simulink subsystem "segment_24S2P"  (R2019b)
settings: Solver=VariableStepAuto  StartTime=0.0  StopTime=10.0  RelTol=1e-3
values from neighbouring files (symbols this model uses):
  cell_prop = struct    [data_load.m]    (also in extend_model_ini.m = data_load('Cell_data.xlsx'))
libraries: fl_lib x44
settings Model: Creator=ZHOU Jinhan  LastModifiedBy=ZHOU Jinhan

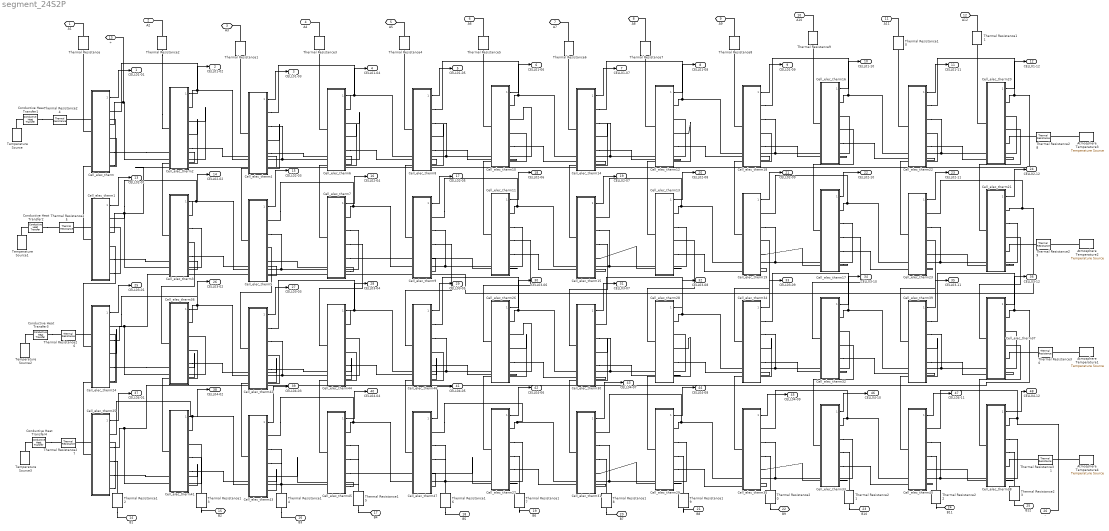
== system segment_24S2P ==
  Atmosphere Temperature{1..4} (4 alike) : fl_lib/Thermal/Thermal Sources/Temperature Source  temperature=cell_prop.T_ext K
      settings: SourceProductName=Simscape
  Cell_elec_therm{,1..47} (48 alike) : Subsystem  ReferencedSubsystem=Cell_elec_therm
  Conductive Heat Transfer{1..4} (4 alike) : fl_lib/Thermal/Thermal Elements/Conductive Heat Transfer  area=0.1 m^2  thickness=0.1 m  th_cond=cell_prop.CFM*0.56657223796 W/(m*K)  T_specify=off  T_priority=None  T=0 K  T_nominal_specify=off  T_nominal_unit=K  T_nominal_value=1  Q_specify=off  Q_priority=None  Q=0 W  Q_nominal_specify=off  Q_nominal_unit=W  Q_nominal_value=1
      settings: SourceProductName=Simscape
  Temperature Source{,1..3} (4 alike) : fl_lib/Thermal/Thermal Sources/Temperature Source  temperature=cell_prop.T_ext K
      settings: SourceProductName=Simscape
  Thermal Resistance{,1..23} (24 alike) : fl_lib/Thermal/Thermal Elements/Thermal Resistance  resistance=1/cell_prop.cell_height*cell_prop.cell_width*cell_prop.wall*0.007874*0.4773 K/W  T_specify=off  T_priority=None  T=0 K  T_nominal_specify=off  T_nominal_unit=K  T_nominal_value=1  Q_specify=off  Q_priority=None  Q=0 W  Q_nominal_specify=off  Q_nominal_unit=W  Q_nominal_value=1
      settings: SourceProductName=Simscape  SourceProductBaseCode=SS
  Thermal Resistance{24..31} (8 alike) : fl_lib/Thermal/Thermal Elements/Thermal Resistance  resistance=1/cell_prop.cell_height*cell_prop.cell_length*cell_prop.wall*0.007874*0.4773 K/W  T_specify=off  T_priority=None  T=0 K  T_nominal_specify=off  T_nominal_unit=K  T_nominal_value=1  Q_specify=off  Q_priority=None  Q=0 W  Q_nominal_specify=off  Q_nominal_unit=W  Q_nominal_value=1
      settings: SourceProductName=Simscape  SourceProductBaseCode=SS
  A1 : PMIOPort  Side=Left
  A2 : PMIOPort  Port=2  Side=Left
  A3 : PMIOPort  Port=3  Side=Left
  A4 : PMIOPort  Port=4  Side=Left
  A5 : PMIOPort  Port=5  Side=Left
  A6 : PMIOPort  Port=6  Side=Left
  A7 : PMIOPort  Port=7  Side=Left
  A8 : PMIOPort  Port=8  Side=Left
  A9 : PMIOPort  Port=9  Side=Left
  A10 : PMIOPort  Port=10  Side=Left
  A11 : PMIOPort  Port=11  Side=Left
  A12 : PMIOPort  Port=12  Side=Left
  + : PMIOPort  Port=13  Side=Left
  B1 : PMIOPort  Port=14  Side=Left
  B2 : PMIOPort  Port=15  Side=Left
  B3 : PMIOPort  Port=16  Side=Left
  B4 : PMIOPort  Port=17  Side=Left
  B5 : PMIOPort  Port=18  Side=Left
  B6 : PMIOPort  Port=19  Side=Left
  B7 : PMIOPort  Port=20  Side=Left
  B8 : PMIOPort  Port=21  Side=Left
  B9 : PMIOPort  Port=22  Side=Left
  B10 : PMIOPort  Port=23  Side=Left
  B11 : PMIOPort  Port=24  Side=Left
  B12 : PMIOPort  Port=25  Side=Left
  - : PMIOPort  Port=26  Side=Left
  CELL01-01 : Outport
  CELL01-02 : Outport  Port=2
  CELL01-03 : Outport  Port=3
  CELL01-04 : Outport  Port=4
  CELL01-05 : Outport  Port=5
  CELL01-06 : Outport  Port=6
  CELL01-07 : Outport  Port=7
  CELL01-08 : Outport  Port=8
  CELL01-09 : Outport  Port=9
  CELL01-10 : Outport  Port=10
  CELL01-11 : Outport  Port=11
  CELL01-12 : Outport  Port=12
  CELL02-01 : Outport  Port=13
  CELL02-02 : Outport  Port=14
  CELL02-03 : Outport  Port=15
  CELL02-04 : Outport  Port=16
  CELL02-05 : Outport  Port=17
  CELL02-06 : Outport  Port=18
  CELL02-07 : Outport  Port=19
  CELL02-08 : Outport  Port=20
  CELL02-09 : Outport  Port=21
  CELL02-10 : Outport  Port=22
  CELL02-11 : Outport  Port=23
  CELL02-12 : Outport  Port=24
  CELL03-01 : Outport  Port=25
  CELL03-02 : Outport  Port=26
  CELL03-03 : Outport  Port=27
  CELL03-04 : Outport  Port=28
  CELL03-05 : Outport  Port=29
  CELL03-06 : Outport  Port=30
  CELL03-07 : Outport  Port=31
  CELL03-08 : Outport  Port=32
  CELL03-09 : Outport  Port=33
  CELL03-10 : Outport  Port=34
  CELL03-11 : Outport  Port=35
  CELL03-12 : Outport  Port=36
  CELL04-01 : Outport  Port=37
  CELL04-02 : Outport  Port=38
  CELL04-03 : Outport  Port=39
  CELL04-04 : Outport  Port=40
  CELL04-05 : Outport  Port=41
  CELL04-06 : Outport  Port=42
  CELL04-07 : Outport  Port=43
  CELL04-08 : Outport  Port=44
  CELL04-09 : Outport  Port=45
  CELL04-10 : Outport  Port=46
  CELL04-11 : Outport  Port=47
  CELL04-12 : Outport  Port=48
  wires:
  Cell_elec_therm3/1 -> CELL02-02/1
  Cell_elec_therm26/1 -> CELL03-06/1
  Cell_elec_therm7/1 -> CELL02-04/1
  Cell_elec_therm28/1 -> CELL03-08/1
  Cell_elec_therm10/1 -> CELL01-06/1
  Cell_elec_therm17/1 -> CELL02-10/1
  Cell_elec_therm32/1 -> CELL03-10/1
  Cell_elec_therm45/1 -> CELL04-04/1
  Cell_elec_therm1/1 -> CELL02-01/1
  Cell_elec_therm9/1 -> CELL02-05/1
  Cell_elec_therm22/1 -> CELL01-11/1
  Cell_elec_therm21/1 -> CELL02-12/1
  Cell_elec_therm15/1 -> CELL02-07/1
  Cell_elec_therm23/1 -> CELL02-11/1
  Cell_elec_therm/1 -> CELL01-01/1
  Cell_elec_therm13/1 -> CELL02-08/1
  Cell_elec_therm20/1 -> CELL01-12/1
  Cell_elec_therm12/1 -> CELL01-08/1
  Cell_elec_therm14/1 -> CELL01-07/1
  Cell_elec_therm18/1 -> CELL01-09/1
  Cell_elec_therm31/1 -> CELL04-07/1
  Cell_elec_therm16/1 -> CELL01-10/1
  Cell_elec_therm19/1 -> CELL02-09/1
  Cell_elec_therm42/1 -> CELL03-03/1
  Cell_elec_therm2/1 -> CELL01-02/1
  Cell_elec_therm25/1 -> CELL04-01/1
  Cell_elec_therm40/1 -> CELL04-11/1
  Cell_elec_therm24/1 -> CELL03-01/1
  Cell_elec_therm27/1 -> CELL04-06/1
  Cell_elec_therm47/1 -> CELL04-05/1
  Cell_elec_therm41/1 -> CELL04-02/1
  Cell_elec_therm46/1 -> CELL03-05/1
  Cell_elec_therm30/1 -> CELL03-07/1
  Cell_elec_therm43/1 -> CELL04-03/1
  Cell_elec_therm33/1 -> CELL04-10/1
  Cell_elec_therm29/1 -> CELL04-08/1
  Cell_elec_therm44/1 -> CELL03-04/1
  Cell_elec_therm37/1 -> CELL03-12/1
  Cell_elec_therm35/1 -> CELL04-09/1
  Cell_elec_therm38/1 -> CELL04-12/1
  Cell_elec_therm34/1 -> CELL03-09/1
  Cell_elec_therm39/1 -> CELL03-11/1
  Cell_elec_therm36/1 -> CELL03-02/1
  Cell_elec_therm6/1 -> CELL01-04/1
  Cell_elec_therm5/1 -> CELL02-03/1
  Cell_elec_therm8/1 -> CELL01-05/1
  Cell_elec_therm11/1 -> CELL02-06/1
  Cell_elec_therm4/1 -> CELL01-03/1
  connections:
  Cell_elec_therm37/RConn1 -- Cell_elec_therm25/RConn2 -- Cell_elec_therm41/RConn2 -- Cell_elec_therm39/RConn1
  Cell_elec_therm12/RConn1 -- Cell_elec_therm16/RConn2 -- Cell_elec_therm18/RConn2 -- Cell_elec_therm14/RConn1
  Cell_elec_therm13/RConn1 -- Cell_elec_therm15/RConn1 -- Cell_elec_therm17/RConn2 -- Cell_elec_therm19/RConn2
  Cell_elec_therm41/RConn1 -- Cell_elec_therm25/RConn1 -- Cell_elec_therm45/RConn2 -- Cell_elec_therm43/RConn2
  Cell_elec_therm28/RConn1 -- Cell_elec_therm34/RConn2 -- Cell_elec_therm32/RConn2 -- Cell_elec_therm30/RConn1
  Cell_elec_therm/RConn2 -- Cell_elec_therm2/RConn2 -- +/RConn1
  Cell_elec_therm5/RConn2 -- Cell_elec_therm3/RConn1 -- Cell_elec_therm1/RConn1 -- Cell_elec_therm7/RConn2
  Cell_elec_therm18/RConn1 -- Cell_elec_therm16/RConn1 -- Cell_elec_therm20/RConn2 -- Cell_elec_therm22/RConn2
  Cell_elec_therm37/RConn2 -- Cell_elec_therm32/RConn1 -- Cell_elec_therm34/RConn1 -- Cell_elec_therm39/RConn2
  Cell_elec_therm9/RConn2 -- Cell_elec_therm5/RConn1 -- Cell_elec_therm7/RConn1 -- Cell_elec_therm11/RConn2
  Cell_elec_therm17/RConn1 -- Cell_elec_therm19/RConn1 -- Cell_elec_therm21/RConn2 -- Cell_elec_therm23/RConn2
  Cell_elec_therm47/RConn2 -- Cell_elec_therm43/RConn1 -- Cell_elec_therm45/RConn1 -- Cell_elec_therm27/RConn2
  Cell_elec_therm1/RConn2 -- Cell_elec_therm20/RConn1 -- Cell_elec_therm22/RConn1 -- Cell_elec_therm3/RConn2
  Cell_elec_therm42/RConn2 -- Cell_elec_therm44/RConn2 -- Cell_elec_therm24/RConn1 -- Cell_elec_therm36/RConn1
  Cell_elec_therm27/RConn1 -- Cell_elec_therm29/RConn2 -- Cell_elec_therm31/RConn2 -- Cell_elec_therm47/RConn1
  Cell_elec_therm35/RConn2 -- Cell_elec_therm31/RConn1 -- Cell_elec_therm29/RConn1 -- Cell_elec_therm33/RConn2
  Cell_elec_therm2/RConn1 -- Cell_elec_therm6/RConn2 -- Cell_elec_therm4/RConn2 -- Cell_elec_therm/RConn1
  Cell_elec_therm6/RConn1 -- Cell_elec_therm10/RConn2 -- Cell_elec_therm8/RConn2 -- Cell_elec_therm4/RConn1
  Cell_elec_therm33/RConn1 -- Cell_elec_therm38/RConn2 -- Cell_elec_therm40/RConn2 -- Cell_elec_therm35/RConn1
  Cell_elec_therm21/RConn1 -- Cell_elec_therm36/RConn2 -- Cell_elec_therm24/RConn2 -- Cell_elec_therm23/RConn1
  Cell_elec_therm10/RConn1 -- Cell_elec_therm12/RConn2 -- Cell_elec_therm14/RConn2 -- Cell_elec_therm8/RConn1
  Cell_elec_therm11/RConn1 -- Cell_elec_therm9/RConn1 -- Cell_elec_therm13/RConn2 -- Cell_elec_therm15/RConn2
  Cell_elec_therm40/RConn1 -- Cell_elec_therm38/RConn1 -- -/RConn1
  Cell_elec_therm28/RConn2 -- Cell_elec_therm46/RConn1 -- Cell_elec_therm26/RConn1 -- Cell_elec_therm30/RConn2
  Cell_elec_therm46/RConn2 -- Cell_elec_therm42/RConn1 -- Cell_elec_therm44/RConn1 -- Cell_elec_therm26/RConn2
  Thermal Resistance3/RConn1 -- A4/RConn1
  Cell_elec_therm12/LConn1 -- Thermal Resistance7/LConn1
  Cell_elec_therm7/RConn4 -- Cell_elec_therm9/RConn5
  Cell_elec_therm3/RConn4 -- Cell_elec_therm5/RConn5
  Cell_elec_therm17/RConn5 -- Cell_elec_therm19/RConn4
  Cell_elec_therm7/RConn5 -- Cell_elec_therm5/RConn4
  Cell_elec_therm10/LConn1 -- Thermal Resistance5/LConn1
  Cell_elec_therm45/LConn1 -- Cell_elec_therm44/RConn3
  Cell_elec_therm15/RConn3 -- Cell_elec_therm30/LConn1
  Cell_elec_therm10/RConn4 -- Cell_elec_therm14/RConn5
  Cell_elec_therm21/RConn5 -- Cell_elec_therm23/RConn4
  Thermal Resistance23/LConn1 -- B12/RConn1
  Cell_elec_therm13/RConn5 -- Cell_elec_therm15/RConn4
  Cell_elec_therm46/RConn4 -- Cell_elec_therm26/RConn5
  Cell_elec_therm22/RConn4 -- Cell_elec_therm20/RConn5
  Cell_elec_therm6/RConn4 -- Cell_elec_therm8/RConn5
  Cell_elec_therm33/LConn1 -- Cell_elec_therm32/RConn3
  Cell_elec_therm21/LConn1 -- Cell_elec_therm20/RConn3
  Cell_elec_therm29/LConn1 -- Cell_elec_therm28/RConn3
  Cell_elec_therm16/RConn4 -- Cell_elec_therm22/RConn5
  Cell_elec_therm23/LConn1 -- Cell_elec_therm22/RConn3
  Thermal Resistance2/LConn1 -- Cell_elec_therm2/LConn1
  Cell_elec_therm17/RConn3 -- Cell_elec_therm32/LConn1
  Cell_elec_therm1/LConn1 -- Cell_elec_therm/RConn3
  Cell_elec_therm32/RConn4 -- Cell_elec_therm39/RConn5
  Cell_elec_therm39/RConn4 -- Cell_elec_therm37/RConn5
  Cell_elec_therm14/RConn4 -- Cell_elec_therm12/RConn5
  Atmosphere Temperature4/LConn1 -- Thermal Resistance31/LConn1
  Cell_elec_therm37/LConn1 -- Cell_elec_therm21/RConn3
  Cell_elec_therm44/RConn4 -- Cell_elec_therm46/RConn5
  Cell_elec_therm17/LConn1 -- Cell_elec_therm16/RConn3
  Cell_elec_therm13/LConn1 -- Cell_elec_therm12/RConn3
  Cell_elec_therm15/LConn1 -- Cell_elec_therm14/RConn3
  Thermal Resistance9/RConn1 -- A10/RConn1
  Cell_elec_therm9/RConn3 -- Cell_elec_therm46/LConn1
  Cell_elec_therm18/RConn4 -- Cell_elec_therm16/RConn5
  Conductive Heat Transfer4/RConn1 -- Thermal Resistance27/RConn1
  Cell_elec_therm19/LConn1 -- Cell_elec_therm18/RConn3
  Cell_elec_therm22/LConn1 -- Thermal Resistance10/LConn1
  Cell_elec_therm34/LConn1 -- Cell_elec_therm19/RConn3
  Cell_elec_therm27/RConn4 -- Cell_elec_therm31/RConn5
  Cell_elec_therm17/RConn4 -- Cell_elec_therm23/RConn5
  Cell_elec_therm25/RConn4 -- Cell_elec_therm41/RConn5
  Cell_elec_therm11/RConn5 -- Cell_elec_therm9/RConn4
  Thermal Resistance6/RConn1 -- A7/RConn1
  Cell_elec_therm27/LConn1 -- Cell_elec_therm26/RConn3
  Cell_elec_therm/RConn4 -- Cell_elec_therm2/RConn5
  Cell_elec_therm28/RConn4 -- Cell_elec_therm34/RConn5
  Cell_elec_therm27/RConn5 -- Cell_elec_therm47/RConn4
  Cell_elec_therm24/LConn1 -- Cell_elec_therm1/RConn3
  Cell_elec_therm30/RConn4 -- Cell_elec_therm28/RConn5
  Cell_elec_therm36/RConn4 -- Cell_elec_therm42/RConn5
  Cell_elec_therm41/LConn1 -- Cell_elec_therm36/RConn3
  Atmosphere Temperature3/LConn1 -- Thermal Resistance28/LConn1
  Cell_elec_therm42/LConn1 -- Cell_elec_therm5/RConn3
  Cell_elec_therm43/LConn1 -- Cell_elec_therm42/RConn3
  Cell_elec_therm47/LConn1 -- Cell_elec_therm46/RConn3
  Cell_elec_therm33/RConn4 -- Cell_elec_therm40/RConn5
  Cell_elec_therm35/LConn1 -- Cell_elec_therm34/RConn3
  Cell_elec_therm28/LConn1 -- Cell_elec_therm13/RConn3
  Cell_elec_therm26/RConn4 -- Cell_elec_therm30/RConn5
  Cell_elec_therm38/RConn5 -- Cell_elec_therm40/RConn4
  Cell_elec_therm24/RConn4 -- Cell_elec_therm36/RConn5
  Cell_elec_therm34/RConn4 -- Cell_elec_therm32/RConn5
  Cell_elec_therm36/LConn1 -- Cell_elec_therm3/RConn3
  Cell_elec_therm25/LConn1 -- Cell_elec_therm24/RConn3
  Cell_elec_therm38/LConn1 -- Cell_elec_therm37/RConn3
  Cell_elec_therm41/RConn4 -- Cell_elec_therm43/RConn5
  Cell_elec_therm31/LConn1 -- Cell_elec_therm30/RConn3
  Cell_elec_therm42/RConn4 -- Cell_elec_therm44/RConn5
  Cell_elec_therm45/RConn5 -- Cell_elec_therm43/RConn4
  Cell_elec_therm29/RConn5 -- Cell_elec_therm31/RConn4
  Cell_elec_therm45/RConn4 -- Cell_elec_therm47/RConn5
  Cell_elec_therm33/RConn5 -- Cell_elec_therm35/RConn4
  Cell_elec_therm29/RConn4 -- Cell_elec_therm35/RConn5
  Cell_elec_therm40/LConn1 -- Cell_elec_therm39/RConn3
  Cell_elec_therm2/RConn4 -- Cell_elec_therm4/RConn5
  Cell_elec_therm11/LConn1 -- Cell_elec_therm10/RConn3
  Cell_elec_therm8/RConn4 -- Cell_elec_therm10/RConn5
  Thermal Resistance1/RConn1 -- A3/RConn1
  Cell_elec_therm18/LConn1 -- Thermal Resistance8/LConn1
  Cell_elec_therm5/LConn1 -- Cell_elec_therm4/RConn3
  Cell_elec_therm7/LConn1 -- Cell_elec_therm6/RConn3
  Thermal Resistance21/LConn1 -- B10/RConn1
  Cell_elec_therm12/RConn4 -- Cell_elec_therm18/RConn5
  Cell_elec_therm9/LConn1 -- Cell_elec_therm8/RConn3
  Cell_elec_therm4/RConn4 -- Cell_elec_therm6/RConn5
  Cell_elec_therm7/RConn3 -- Cell_elec_therm44/LConn1
  Cell_elec_therm1/RConn4 -- Cell_elec_therm3/RConn5
  Cell_elec_therm11/RConn4 -- Cell_elec_therm15/RConn5
  Cell_elec_therm39/LConn1 -- Cell_elec_therm23/RConn3
  Cell_elec_therm11/RConn3 -- Cell_elec_therm26/LConn1
  Cell_elec_therm13/RConn4 -- Cell_elec_therm19/RConn5
  Cell_elec_therm3/LConn1 -- Cell_elec_therm2/RConn3
  Atmosphere Temperature2/LConn1 -- Thermal Resistance29/LConn1
  Thermal Resistance11/RConn1 -- A12/RConn1
  Cell_elec_therm47/RConn3 -- Thermal Resistance16/RConn1
  Thermal Resistance12/LConn1 -- B1/RConn1
  Thermal Resistance17/LConn1 -- B6/RConn1
  Thermal Resistance15/LConn1 -- B4/RConn1
  Thermal Resistance22/LConn1 -- B11/RConn1
  Atmosphere Temperature1/LConn1 -- Thermal Resistance30/LConn1
  Cell_elec_therm43/RConn3 -- Thermal Resistance14/RConn1
  Thermal Resistance18/LConn1 -- B7/RConn1
  Cell_elec_therm29/RConn3 -- Thermal Resistance19/RConn1
  Thermal Resistance13/LConn1 -- B2/RConn1
  Thermal Resistance20/LConn1 -- B9/RConn1
  Thermal Resistance4/RConn1 -- A5/RConn1
  Conductive Heat Transfer1/RConn1 -- Thermal Resistance24/RConn1
  Cell_elec_therm/LConn1 -- Thermal Resistance/LConn1
  Cell_elec_therm1/RConn5 -- Thermal Resistance25/LConn1
  Thermal Resistance/RConn1 -- A1/RConn1
  Thermal Resistance2/RConn1 -- A2/RConn1
  Cell_elec_therm4/LConn1 -- Thermal Resistance1/LConn1
  Cell_elec_therm6/LConn1 -- Thermal Resistance3/LConn1
  Cell_elec_therm8/LConn1 -- Thermal Resistance4/LConn1
  Thermal Resistance5/RConn1 -- A6/RConn1
  Cell_elec_therm14/LConn1 -- Thermal Resistance6/LConn1
  Thermal Resistance7/RConn1 -- A8/RConn1
  Thermal Resistance8/RConn1 -- A9/RConn1
  Cell_elec_therm16/LConn1 -- Thermal Resistance9/LConn1
  Thermal Resistance10/RConn1 -- A11/RConn1
  Cell_elec_therm20/LConn1 -- Thermal Resistance11/LConn1
  Cell_elec_therm25/RConn3 -- Thermal Resistance12/RConn1
  Cell_elec_therm41/RConn3 -- Thermal Resistance13/RConn1
  Thermal Resistance14/LConn1 -- B3/RConn1
  Cell_elec_therm45/RConn3 -- Thermal Resistance15/RConn1
  Thermal Resistance16/LConn1 -- B5/RConn1
  Cell_elec_therm27/RConn3 -- Thermal Resistance17/RConn1
  Cell_elec_therm31/RConn3 -- Thermal Resistance18/RConn1
  Thermal Resistance19/LConn1 -- B8/RConn1
  Cell_elec_therm35/RConn3 -- Thermal Resistance20/RConn1
  Cell_elec_therm33/RConn3 -- Thermal Resistance21/RConn1
  Cell_elec_therm40/RConn3 -- Thermal Resistance22/RConn1
  Cell_elec_therm38/RConn3 -- Thermal Resistance23/RConn1
  Cell_elec_therm/RConn5 -- Thermal Resistance24/LConn1
  Conductive Heat Transfer2/RConn1 -- Thermal Resistance25/RConn1
  Cell_elec_therm24/RConn5 -- Thermal Resistance26/LConn1
  Cell_elec_therm25/RConn5 -- Thermal Resistance27/LConn1
  Cell_elec_therm20/RConn4 -- Thermal Resistance28/RConn1
  Cell_elec_therm21/RConn4 -- Thermal Resistance29/RConn1
  Cell_elec_therm37/RConn4 -- Thermal Resistance30/RConn1
  Cell_elec_therm38/RConn4 -- Thermal Resistance31/RConn1
  Conductive Heat Transfer1/LConn1 -- Temperature Source/LConn1
  Conductive Heat Transfer2/LConn1 -- Temperature Source1/LConn1
  Conductive Heat Transfer3/LConn1 -- Temperature Source2/LConn1
  Conductive Heat Transfer4/LConn1 -- Temperature Source3/LConn1
  Conductive Heat Transfer3/RConn1 -- Thermal Resistance26/RConn1
